simulink library "csu_kfd_orb_feature_matching_lib"  (R2014b)
settings: Solver=ode45  StartTime=0.0  StopTime=10.0  RelTol=1e-3
undefined symbols (not defined in the file): cam_kir_image_size
libraries: util_info_lib x1
settings Model: Creator=escrane  LastModifiedBy=mstewart

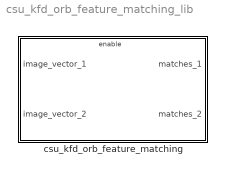
== system csu_kfd_orb_feature_matching_lib ==
  csu_kfd_orb_feature_matching : Subsystem  mask{size=cam_kir_image_size}
      mask prompts: size "Image Size [cols rows]"

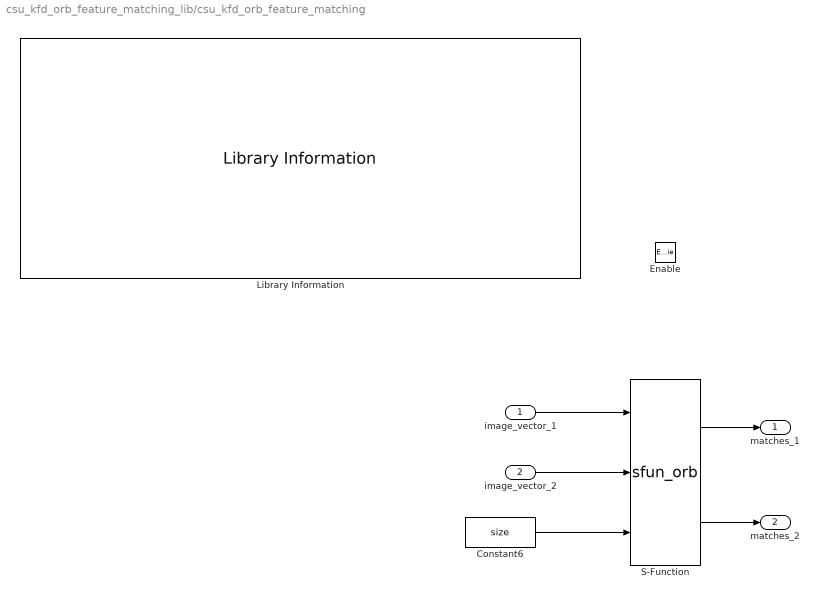
== system csu_kfd_orb_feature_matching_lib/csu_kfd_orb_feature_matching ==
  image_vector_1 : Inport
  image_vector_2 : Inport  Port=2
  Enable : EnablePort
  Constant6 : Constant  Value=size
  Library Information : util_info_lib/Library Information  owner='NONE'
  S-Function : S-Function  FunctionName=sfun_orb  Parameters=100  EnableBusSupport=off
  matches_1 : Outport
  matches_2 : Outport  Port=2
  wires:
  S-Function/1 -> matches_1/1
  S-Function/2 -> matches_2/1
  image_vector_1/1 -> S-Function/1
  image_vector_2/1 -> S-Function/2
  Constant6/1 -> S-Function/3
